simulink model "MSDR_v1.1"  (R2018a)
settings: Solver=ode3  StartTime=0.0  StopTime=21600  FixedStep=0.05
values from neighbouring files (symbols this model uses):
  a_f = -3.22E-5    (= -3.22e-05)    [MSDR_parameters.m]
  a_g = +2.35E-5    (= 2.35e-05)    [MSDR_parameters.m]
  A_s = 1.2245    [MSDR_parameters.m]
  beta = [0.000223, 0.001457, 0.001307, 0.002628, 0.000766, 0.000280]    [MSDR_parameters.m]
  beta_t = sum(beta)    [MSDR_parameters.m]
  ce1 = 1.2471e-07    [MSDR_parameters.m]
  ce2 = 5.3816e-14    [MSDR_parameters.m]
  ce3 = 3.3721e-08    [MSDR_parameters.m]
  Cp_fw = 3200.448e-6    (= 0.003200448)    [MSDR_parameters.m]
  Cp_hr = 0.0021520    (= 0.002152)    [MSDR_parameters.m]
  Cp_p = Cp_s_shx    (= 0.00154912)    [MSDR_parameters.m]
  Cp_s = Cp_s*1e-6    (= 3.588208e-09)    [MSDR_parameters.m]
  Cp_s_shx = 1549.12e-6    (= 0.00154912)    [MSDR_parameters.m]
  Cp_sc = 4761.392e-6    (= 0.004761392)    [MSDR_parameters.m]
  Cp_w = 456.056e-6    (= 0.000456056)    [MSDR_parameters.m]
  D_it = 0.0141478    [MSDR_parameters.m]
  D_ot = 0.015875    [MSDR_parameters.m]
  dHs_dPs = -0.042433622114357    (= -0.0424336221144)    [MSDR_parameters.m]
  eta_hp_isen = 0.861    [MSDR_parameters.m]
  eta_lp_isen = 0.861    [MSDR_parameters.m]
  gamma_I = 5.1135e-2    (= 0.051135)    [MSDR_parameters.m]
  gamma_Xe = 1.1628e-2    (= 0.011628)    [MSDR_parameters.m]
  H_fwh1 = 0.46009    [MSDR_parameters.m]
  h_fwh1 = 0.5927    [MSDR_parameters.m]
  H_fwh2 = 0.6784    [MSDR_parameters.m]
  h_fwh2 = 0.5927    [MSDR_parameters.m]
  H_lp_isen = 958.4*1054.35e-6/0.45359237    (= 2.22774699671)    [MSDR_parameters.m]
  H_nc = 3.2952    [MSDR_parameters.m]
  h_pw = h_s_shx    (= 0.00567446)    [MSDR_parameters.m]
  H_rh = 2.8115    [MSDR_parameters.m]
  h_wb = 13349.334646671E-6    (= 0.0133493346467)    [MSDR_parameters.m]
  h_ws = 5732.378387768E-6    (= 0.00573237838777)    [MSDR_parameters.m]
  h_wsc = 8385.005556375E-6    (= 0.00838500555638)    [MSDR_parameters.m]
  hA_fg = [h_fg*A_fg/2, h_fg*A_fg/2]    [MSDR_parameters.m]
  hA_p_phx1 = h_p_phx*A_p_phx    [MSDR_parameters.m]
  hA_p_phx2 = h_p_phx*A_p_phx    [MSDR_parameters.m]
  hA_p_phx3 = h_p_phx*A_p_phx    [MSDR_parameters.m]
  hA_p_phx4 = h_p_phx*A_p_phx    [MSDR_parameters.m]
  hA_p_phx5 = h_p_phx*A_p_phx    [MSDR_parameters.m]
  hA_p_phx6 = h_p_phx*A_p_phx    [MSDR_parameters.m]
  hA_p_shx1 = h_p_shx*A_p_shx    [MSDR_parameters.m]
  hA_p_shx2 = h_p_shx*A_p_shx    [MSDR_parameters.m]
  hA_p_shx3 = h_p_shx*A_p_shx    [MSDR_parameters.m]
  hA_p_shx4 = h_p_shx*A_p_shx    [MSDR_parameters.m]
  hA_p_shx5 = h_p_shx*A_p_shx    [MSDR_parameters.m]
  hA_p_shx6 = h_p_shx*A_p_shx    [MSDR_parameters.m]
  hA_s_phx1 = h_s_phx*A_s_phx    [MSDR_parameters.m]
  hA_s_phx2 = h_s_phx*A_s_phx    [MSDR_parameters.m]
  hA_s_phx3 = h_s_phx*A_s_phx    [MSDR_parameters.m]
  hA_s_phx4 = h_s_phx*A_s_phx    [MSDR_parameters.m]
  hA_s_phx5 = h_s_phx*A_s_phx    [MSDR_parameters.m]
  hA_s_phx6 = h_s_phx*A_s_phx    [MSDR_parameters.m]
  hA_s_shx1 = h_s_shx*A_s_shx    [MSDR_parameters.m]
  hA_s_shx2 = h_s_shx*A_s_shx    [MSDR_parameters.m]
  hA_s_shx3 = h_s_shx*A_s_shx    [MSDR_parameters.m]
  hA_s_shx4 = h_s_shx*A_s_shx    [MSDR_parameters.m]
  hA_s_shx5 = h_s_shx*A_s_shx    [MSDR_parameters.m]
  hA_s_shx6 = h_s_shx*A_s_shx    [MSDR_parameters.m]
  I_0 = gamma_I*Sig_f_msdr*phi_0/lam_I    (= 4.38204721773e+16)    [MSDR_parameters.m]
  Ifa = [0.25, 0.25]    [MSDR_parameters.m]
  Ifb = [0.25, 0.25]    [MSDR_parameters.m]
  Ig = [0.5, 0.5]    [MSDR_parameters.m]
  K_1 = 11.632248097704855    (= 11.6322480977)    [MSDR_parameters.m]
  K_4 = b(1)    [MSDR_parameters.m]
  K_5 = a(1)    [MSDR_parameters.m]
  K_b = 12.834854076292217    (= 12.8348540763)    [MSDR_parameters.m]
  K_b_hp = 0.1634    [MSDR_parameters.m]
  K_b_lp = 0.2174    [MSDR_parameters.m]
  K_sc = -17.615718797133468    (= -17.6157187971)    [MSDR_parameters.m]
  ka = [0.235, 0.235]    [MSDR_parameters.m]
  kb = [0.235, 0.235]    [MSDR_parameters.m]
  kga = [0.015, 0.015]    [MSDR_parameters.m]
  kgb = [0.015, 0.015]    [MSDR_parameters.m]
  L = 8.5344    [MSDR_parameters.m]
  L_b = 2.3645    [MSDR_parameters.m]
  L_s = 4.723    [MSDR_parameters.m]
  Lam = 2.400E-04    (= 0.00024)    [MSDR_parameters.m]
  lam = [0.0124, 0.0305, 0.111, 0.301, 1.14, 3.01]    [MSDR_parameters.m]
  lam_bubl = 2.0e-2    (= 0.02)    [MSDR_parameters.m]
  lam_I = 2.875e-5    (= 2.875e-05)    [MSDR_parameters.m]
  lam_Xe = 2.0916e-5    (= 2.0916e-05)    [MSDR_parameters.m]
  m_3m = W_3*2    (= 8618.207327)    [MSDR_parameters.m]
  m_fm = W_f*2    (= 9978.96)    [MSDR_parameters.m]
  m_sb = 1717    [MSDR_parameters.m]
  M_stm = 0.018    [MSDR_parameters.m]
  mb_cpb = 2.689619410657651e+00    (= 2.68961941066)    [MSDR_parameters.m]
  mcp_fa = mfa*Cp_f    [MSDR_parameters.m]
  mcp_fb = mfb*Cp_f    [MSDR_parameters.m]
  mcp_g = mg*Cp_g    [MSDR_parameters.m]
  mcp_p_phx1 = Cp_p_phx*mp_phx1    [MSDR_parameters.m]
  mcp_p_phx2 = Cp_p_phx*mp_phx2    [MSDR_parameters.m]
  mcp_p_phx3 = Cp_p_phx*mp_phx3    [MSDR_parameters.m]
  mcp_p_phx4 = Cp_p_phx*mp_phx4    [MSDR_parameters.m]
  mcp_p_phx5 = Cp_p_phx*mp_phx5    [MSDR_parameters.m]
  mcp_p_phx6 = Cp_p_phx*mp_phx6    [MSDR_parameters.m]
  mcp_p_shx1 = Cp_p_shx*mp_shx1    [MSDR_parameters.m]
  mcp_p_shx2 = Cp_p_shx*mp_shx2    [MSDR_parameters.m]
  mcp_p_shx3 = Cp_p_shx*mp_shx3    [MSDR_parameters.m]
  mcp_p_shx4 = Cp_p_shx*mp_shx4    [MSDR_parameters.m]
  mcp_p_shx5 = Cp_p_shx*mp_shx5    [MSDR_parameters.m]
  mcp_p_shx6 = Cp_p_shx*mp_shx6    [MSDR_parameters.m]
  mcp_s_phx1 = Cp_s_phx*ms_phx1    [MSDR_parameters.m]
  mcp_s_phx2 = Cp_s_phx*ms_phx2    [MSDR_parameters.m]
  mcp_s_phx3 = Cp_s_phx*ms_phx3    [MSDR_parameters.m]
  mcp_s_phx4 = Cp_s_phx*ms_phx4    [MSDR_parameters.m]
  mcp_s_phx5 = Cp_s_phx*ms_phx5    [MSDR_parameters.m]
  mcp_s_phx6 = Cp_s_phx*ms_phx6    [MSDR_parameters.m]
  mcp_s_shx1 = Cp_s_shx*ms_shx1    [MSDR_parameters.m]
  mcp_s_shx2 = Cp_s_shx*ms_shx1    [MSDR_parameters.m]
  mcp_s_shx3 = Cp_s_shx*ms_shx1    [MSDR_parameters.m]
  mcp_s_shx4 = Cp_s_shx*ms_shx1    [MSDR_parameters.m]
  mcp_s_shx5 = Cp_s_shx*ms_shx1    [MSDR_parameters.m]
  mcp_s_shx6 = Cp_s_shx*ms_shx1    [MSDR_parameters.m]
  mcp_t_phx1 = Cp_t_phx*mt_phx1    [MSDR_parameters.m]
  mcp_t_phx2 = Cp_t_phx*mt_phx2    [MSDR_parameters.m]
  mcp_t_phx3 = Cp_t_phx*mt_phx3    [MSDR_parameters.m]
  mcp_t_phx4 = Cp_t_phx*mt_phx4    [MSDR_parameters.m]
  mcp_t_phx5 = Cp_t_phx*mt_phx5    [MSDR_parameters.m]
  mcp_t_phx6 = Cp_t_phx*mt_phx6    [MSDR_parameters.m]
  mcp_t_shx1 = Cp_t_phx*mt_shx1    [MSDR_parameters.m]
  ... (+177 more)
undefined symbols (not defined in the file or in its folder): C0, H_rh_table, H_rh_table1, H_rh_table2, H_rhvap_table, H_s_table, H_table, hA_p_thx1, hA_p_thx2, hA_p_thx3, hA_s_thx1, hA_s_thx2, hA_s_thx3, mcp_p_thx1, mcp_p_thx2, mcp_p_thx3, mcp_s_thx1, mcp_s_thx2, mcp_s_thx3, mcp_t_thx1, mcp_t_thx2, mcp_t_thx3, mp_thx1, mp_thx2, mp_thx3, ms_thx1, ms_thx2, ms_thx3, P_nc_table, P_rh_table, P_rh_table1, pres_table, rho_rh_table, rho_table, SV_nc_table, T0_p_thx1, T0_p_thx2, T0_p_thx3, T0_s_thx1, T0_s_thx2, T0_s_thx3, T0_t_thx1, T0_t_thx2, T0_t_thx3, temp_table, u14, Wp_thx1, Wp_thx2
libraries: simulink x13
(part 2 of 6)

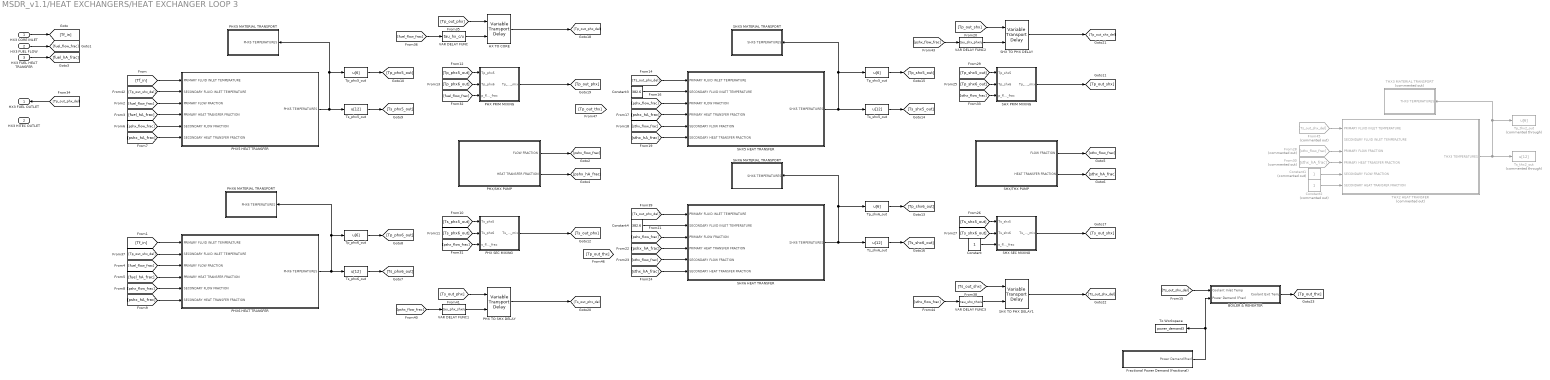
== system MSDR_v1.1/HEAT EXCHANGERS/HEAT EXCHANGER LOOP 3 ==
  HX3 CORE INLET : Inport
  HX3 FUEL FLOW : Inport  Port=2
  HX3 FUEL HEAT TRANSFER : Inport  Port=3
  BOILER & REHEATER : Subsystem
  Constant : Constant
  Constant1 : Constant  Commented=on
  Constant2 : Constant  Commented=on
  Constant3 : Constant  Value=382.6
  Constant4 : Constant  Value=382.6
  Fractional Power Demand (fractional) : Subsystem
  From28 : From  Commented=on  GotoTag=sthx_flow_frac
  From30 : From  Commented=on  GotoTag=sthx_hA_frac
  From45 : From  Commented=on  GotoTag=Ts_out_shx_del
  HX TO CORE : VariableTransportDelay  MaximumDelay=1000000000000  InitialOutput=T0_p_phx5(4)
  PHX PRIM MIXING : Subsystem
  PHX SEC MIXING : Subsystem
  PHX TO SHX DELAY : VariableTransportDelay  MaximumDelay=100000000000  InitialOutput=T0_s_phx5(4)
  PHX/SHX PUMP : Subsystem
  PHX5 HEAT TRANSFER : Subsystem
  PHX5 MATERIAL TRANSPORT : Subsystem
  PHX6 HEAT TRANSFER : Subsystem
  PHX6 MATERIAL TRANSPORT : Subsystem
  SHX PRIM MIXING : Subsystem
  SHX SEC MIXING : Subsystem
  SHX TO PHX DELAY : VariableTransportDelay  MaximumDelay=1000000000000  InitialOutput=T0_p_shx5(4)
  SHX TO PHX DELAY1 : VariableTransportDelay  MaximumDelay=1000000000000  InitialOutput=T0_s_shx5(4)
  SHX/THX PUMP : Subsystem
  SHX5 HEAT TRANSFER : Subsystem
  SHX5 MATERIAL TRANSPORT : Subsystem
  SHX6 HEAT TRANSFER : Subsystem
  SHX6 MATERIAL TRANSPORT : Subsystem
  THX2 HEAT TRANSFER : Subsystem  Commented=on
  THX3 MATERIAL TRANSPORT : Subsystem  Commented=on
  To Workspace : ToWorkspace  VariableName=power_demand3  SampleTime=-1
  Tp_phx5_out : Fcn  Expr=u[6]
  Tp_phx6_out : Fcn  Expr=u[6]
  Tp_shx5_out : Fcn  Expr=u[6]
  Tp_shx6_out : Fcn  Expr=u[6]
  Tp_thx2_out : Fcn  Commented=through  Expr=u[6]
  Ts_phx5_out : Fcn  Expr=u[12]
  Ts_phx6_out : Fcn  Expr=u[12]
  Ts_shx5_out : Fcn  Expr=u[12]
  Ts_shx6_out : Fcn  Expr=u[12]
  Ts_thx2_out : Fcn  Commented=through  Expr=u[12]
  VAR DELAY FUNC : Fcn  Expr=tau_hx_c/u
  VAR DELAY FUNC1 : Fcn  Expr=tau_phx_shx/u
  VAR DELAY FUNC2 : Fcn  Expr=tau_shx_phx/u
  VAR DELAY FUNC3 : Fcn  Expr=tau_shx_thx/u
  HX3 FUEL OUTLET : Outport
  HX3 HITEC OUTLET : Outport  Port=2
  wires:
  HX3 FUEL FLOW/1 -> [fuel_flow_frac]
  HX3 FUEL HEAT TRANSFER/1 -> [fuel_hA_frac]
  HX3 CORE INLET/1 -> [Tf_in]
  [Tp_out_phx_del] -> HX3 FUEL OUTLET/1
  PHX5 HEAT TRANSFER/1(PHX5 TEMPERATURES) -> PHX5 MATERIAL TRANSPORT/1(PHX5 TEMPERATURES), Tp_phx5_out/1, Ts_phx5_out/1
  Tp_phx5_out/1 -> [Tp_phx5_out]
  Ts_phx5_out/1 -> [Ts_phx5_out]
  PHX6 HEAT TRANSFER/1(PHX6 TEMPERATURES) -> PHX6 MATERIAL TRANSPORT/1(PHX6 TEMPERATURES), Tp_phx6_out/1, Ts_phx6_out/1
  Tp_phx6_out/1 -> [Tp_phx6_out]
  Ts_phx6_out/1 -> [Ts_phx6_out]
  PHX/SHX PUMP/2(HEAT TRANSFER FRACTION) -> [pshx_hA_frac]
  [pshx_flow_frac] -> PHX SEC MIXING/3(s_flow_frac)
  [Ts_phx5_out] -> PHX SEC MIXING/1(Ts_phx5)
  PHX/SHX PUMP/1(FLOW FRACTION) -> [pshx_flow_frac]
  [Ts_phx6_out] -> PHX SEC MIXING/2(Ts_phx6)
  PHX SEC MIXING/1(Ts_phx_mix) -> [Ts_out_phx]
  [Tp_phx6_out] -> PHX PRIM MIXING/2(Tp_phx6)
  PHX PRIM MIXING/1(Tp_phx_mix) -> [Tp_out_phx]
  [Tp_phx5_out] -> PHX PRIM MIXING/1(Tp_phx5)
  [fuel_flow_frac] -> PHX PRIM MIXING/3(p_flow_frac)
  Ts_shx5_out/1 -> [Ts_shx5_out]
  Tp_shx5_out/1 -> [Tp_shx5_out]
  SHX5 HEAT TRANSFER/1(SHX5 TEMPERATURES) -> Ts_shx5_out/1, SHX5 MATERIAL TRANSPORT/1(SHX5 TEMPERATURES), Tp_shx5_out/1
  SHX6 HEAT TRANSFER/1(SHX6 TEMPERATURES) -> Ts_shx6_out/1, SHX6 MATERIAL TRANSPORT/1(SHX6 TEMPERATURES), Tp_shx6_out/1
  Ts_shx6_out/1 -> [Ts_shx6_out]
  Tp_shx6_out/1 -> [Tp_shx6_out]
  SHX/THX PUMP/1(FLOW FRACTION) -> [sthx_flow_frac]
  [sthx_flow_frac] -> SHX PRIM MIXING/3(p_flow_frac)
  SHX SEC MIXING/1(Ts_shx_mix) -> [Ts_out_shx]
  SHX/THX PUMP/2(HEAT TRANSFER FRACTION) -> [sthx_hA_frac]
  SHX PRIM MIXING/1(Tp_shx_mix) -> [Tp_out_shx]
  [Ts_shx5_out] -> SHX SEC MIXING/1(Ts_shx5)
  [Tp_shx5_out] -> SHX PRIM MIXING/1(Tp_shx5)
  Constant/1 -> SHX SEC MIXING/3(s_flow_frac)
  [Ts_shx6_out] -> SHX SEC MIXING/2(Ts_shx6)
  [Tp_shx6_out] -> SHX PRIM MIXING/2(Tp_shx6)
  THX2 HEAT TRANSFER/1(THX3 TEMPERATURES) -> THX3 MATERIAL TRANSPORT/1(THX3 TEMPERATURES), Tp_thx2_out/1, Ts_thx2_out/1
  [pshx_hA_frac] -> PHX5 HEAT TRANSFER/6(SECONDARY HEAT TRANSFER FRACTION)
  [Tp_out_shx_del] -> PHX5 HEAT TRANSFER/2(SECONDARY FLUID INLET TEMPERATURE)
  [pshx_flow_frac] -> PHX5 HEAT TRANSFER/5(SECONDARY FLOW FRACTION)
  [fuel_hA_frac] -> PHX5 HEAT TRANSFER/4(PRIMARY HEAT TRANSFER FRACTION)
  [Tf_in] -> PHX5 HEAT TRANSFER/1(PRIMARY FLUID INLET TEMPERATURE)
  [fuel_flow_frac] -> PHX5 HEAT TRANSFER/3(PRIMARY FLOW FRACTION)
  [pshx_flow_frac] -> PHX6 HEAT TRANSFER/5(SECONDARY FLOW FRACTION)
  [fuel_hA_frac] -> PHX6 HEAT TRANSFER/4(PRIMARY HEAT TRANSFER FRACTION)
  [pshx_hA_frac] -> PHX6 HEAT TRANSFER/6(SECONDARY HEAT TRANSFER FRACTION)
  [Tf_in] -> PHX6 HEAT TRANSFER/1(PRIMARY FLUID INLET TEMPERATURE)
  [fuel_flow_frac] -> PHX6 HEAT TRANSFER/3(PRIMARY FLOW FRACTION)
  [Tp_out_shx_del] -> PHX6 HEAT TRANSFER/2(SECONDARY FLUID INLET TEMPERATURE)
  [fuel_flow_frac] -> VAR DELAY FUNC/1
  [Tp_out_phx] -> HX TO CORE/1
  HX TO CORE/1 -> [Tp_out_phx_del]
  VAR DELAY FUNC/1 -> HX TO CORE/2
  PHX TO SHX DELAY/1 -> [Ts_out_phx_del]
  [pshx_flow_frac] -> VAR DELAY FUNC1/1
  VAR DELAY FUNC1/1 -> PHX TO SHX DELAY/2
  [Ts_out_phx] -> PHX TO SHX DELAY/1
  [pshx_flow_frac] -> SHX5 HEAT TRANSFER/3(PRIMARY FLOW FRACTION)
  [pshx_hA_frac] -> SHX5 HEAT TRANSFER/4(PRIMARY HEAT TRANSFER FRACTION)
  [sthx_hA_frac] -> SHX5 HEAT TRANSFER/6(SECONDARY HEAT TRANSFER FRACTION)
  [Ts_out_phx_del] -> SHX5 HEAT TRANSFER/1(PRIMARY FLUID INLET TEMPERATURE)
  [sthx_flow_frac] -> SHX5 HEAT TRANSFER/5(SECONDARY FLOW FRACTION)
  [sthx_hA_frac] -> SHX6 HEAT TRANSFER/6(SECONDARY HEAT TRANSFER FRACTION)
  [pshx_hA_frac] -> SHX6 HEAT TRANSFER/4(PRIMARY HEAT TRANSFER FRACTION)
  [pshx_flow_frac] -> SHX6 HEAT TRANSFER/3(PRIMARY FLOW FRACTION)
  [sthx_flow_frac] -> SHX6 HEAT TRANSFER/5(SECONDARY FLOW FRACTION)
  [Ts_out_phx_del] -> SHX6 HEAT TRANSFER/1(PRIMARY FLUID INLET TEMPERATURE)
  VAR DELAY FUNC2/1 -> SHX TO PHX DELAY/2
  [Tp_out_shx] -> SHX TO PHX DELAY/1
  [pshx_flow_frac] -> VAR DELAY FUNC2/1
  SHX TO PHX DELAY/1 -> [Tp_out_shx_del]
  [Ts_out_shx] -> SHX TO PHX DELAY1/1
  SHX TO PHX DELAY1/1 -> [Ts_out_shx_del]
  [sthx_flow_frac] -> VAR DELAY FUNC3/1
  VAR DELAY FUNC3/1 -> SHX TO PHX DELAY1/2
  Constant1/1 -> THX2 HEAT TRANSFER/5(SECONDARY FLOW FRACTION)
  Constant2/1 -> THX2 HEAT TRANSFER/6(SECONDARY HEAT TRANSFER FRACTION)
  From45/1 -> THX2 HEAT TRANSFER/1(PRIMARY FLUID INLET TEMPERATURE)
  From28/1 -> THX2 HEAT TRANSFER/3(PRIMARY FLOW FRACTION)
  From30/1 -> THX2 HEAT TRANSFER/4(PRIMARY HEAT TRANSFER FRACTION)
  BOILER & REHEATER/1(Coolant Exit Temp) -> [Tp_out_thx]
  [Ts_out_shx_del] -> BOILER & REHEATER/1(Coolant Inlet Temp)
  Fractional Power Demand (fractional)/1(Power Demand(frac)) -> To Workspace/1, BOILER & REHEATER/2(Power Demand (Frac))
  Constant3/1 -> SHX5 HEAT TRANSFER/2(SECONDARY FLUID INLET TEMPERATURE)
  Constant4/1 -> SHX6 HEAT TRANSFER/2(SECONDARY FLUID INLET TEMPERATURE)

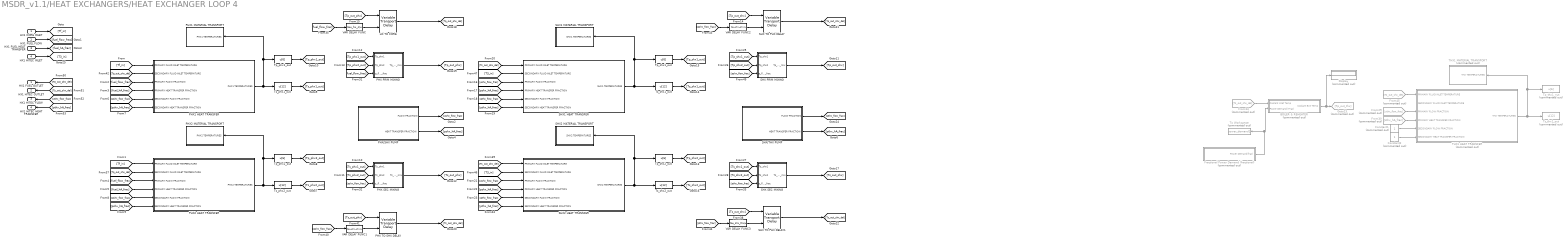
== system MSDR_v1.1/HEAT EXCHANGERS/HEAT EXCHANGER LOOP 4 ==
  HX1 CORE INLET : Inport
  HX1 FUEL FLOW : Inport  Port=2
  HX1 FUEL HEAT TRANSFER : Inport  Port=3
  HX1 HITEC INLET : Inport  Port=4
  BOILER & REHEATER : Subsystem  Commented=on
  Constant1 : Constant  Commented=on
  Constant2 : Constant  Commented=on
  Display : Display  Commented=on
  Fractional Power Demand (fractional) : Subsystem  Commented=on
  From29 : From  Commented=on  GotoTag=sthx_flow_frac
  From30 : From  Commented=on  GotoTag=sthx_hA_frac
  From34 : From  Commented=on  GotoTag=Ts_out_shx_del
  From45 : From  Commented=on  GotoTag=Ts_out_shx_del
  Goto23 : Goto  Commented=on  GotoTag=Tp_out_thx
  HX TO CORE : VariableTransportDelay  MaximumDelay=1000000000000  InitialOutput=T0_p_phx1(4)
  PHX PRIM MIXING : Subsystem
  PHX SEC MIXING : Subsystem
  PHX TO SHX DELAY : VariableTransportDelay  MaximumDelay=100000000000  InitialOutput=T0_s_phx1(4)
  PHX/SHX PUMP : Subsystem
  PHX1 HEAT TRANSFER : Subsystem
  PHX1 MATERIAL TRANSPORT : Subsystem
  PHX2 HEAT TRANSFER : Subsystem
  PHX2 MATERIAL TRANSPORT : Subsystem
  SHX PRIM MIXING : Subsystem
  SHX SEC MIXING : Subsystem
  SHX TO PHX DELAY : VariableTransportDelay  MaximumDelay=1000000000000  InitialOutput=T0_p_shx1(4)
  SHX TO PHX DELAY1 : VariableTransportDelay  MaximumDelay=1000000000000  InitialOutput=T0_s_shx1(4)
  SHX/THX PUMP : Subsystem
  SHX1 HEAT TRANSFER : Subsystem
  SHX1 MATERIAL TRANSPORT : Subsystem
  SHX2 HEAT TRANSFER : Subsystem
  SHX2 MATERIAL TRANSPORT : Subsystem
  THX1 HEAT TRANSFER : Subsystem  Commented=on
  THX1 MATERIAL TRANSPORT : Subsystem  Commented=on
  To Workspace : ToWorkspace  Commented=on  VariableName=power_demand1  SampleTime=-1
  Tp_phx1_out : Fcn  Expr=u[6]
  Tp_phx2_out : Fcn  Expr=u[6]
  Tp_shx1_out : Fcn  Expr=u[6]
  Tp_shx2_out : Fcn  Expr=u[6]
  Tp_thx1_out : Fcn  Commented=on  Expr=u[6]
  Ts_phx1_out : Fcn  Expr=u[12]
  Ts_phx2_out : Fcn  Expr=u[12]
  Ts_shx1_out : Fcn  Expr=u[12]
  Ts_shx2_out : Fcn  Expr=u[12]
  Ts_thx1_out : Fcn  Commented=on  Expr=u[12]
  VAR DELAY FUNC : Fcn  Expr=tau_hx_c/u
  VAR DELAY FUNC1 : Fcn  Expr=tau_phx_shx/u
  VAR DELAY FUNC2 : Fcn  Expr=tau_shx_phx/u
  VAR DELAY FUNC3 : Fcn  Expr=tau_shx_thx/u
  HX1 FUEL OUTLET : Outport
  HX1 HITEC OUTLET : Outport  Port=2
  HX1 HITEC FLOW : Outport  Port=3
  HX1 HITEC HEAT TRANSFER : Outport  Port=4
  wires:
  PHX1 HEAT TRANSFER/1(PHX1 TEMPERATURES) -> PHX1 MATERIAL TRANSPORT/1(PHX1 TEMPERATURES), Tp_phx1_out/1, Ts_phx1_out/1
  THX1 HEAT TRANSFER/1(THX TEMPERATURES) -> THX1 MATERIAL TRANSPORT/1(THX TEMPERATURES), Tp_thx1_out/1, Ts_thx1_out/1
  SHX1 HEAT TRANSFER/1(SHX1 TEMPERATURES) -> Ts_shx1_out/1, Tp_shx1_out/1, SHX1 MATERIAL TRANSPORT/1(SHX1 TEMPERATURES)
  PHX2 HEAT TRANSFER/1(PHX2 TEMPERATURES) -> PHX2 MATERIAL TRANSPORT/1(PHX2 TEMPERATURES), Tp_phx2_out/1, Ts_phx2_out/1
  SHX2 HEAT TRANSFER/1(SHX2 TEMPERATURES) -> Ts_shx2_out/1, SHX2 MATERIAL TRANSPORT/1(SHX2 TEMPERATURES), Tp_shx2_out/1
  HX1 CORE INLET/1 -> [Tf_in]
  [Tf_in] -> PHX1 HEAT TRANSFER/1(PRIMARY FLUID INLET TEMPERATURE)
  [Tf_in] -> PHX2 HEAT TRANSFER/1(PRIMARY FLUID INLET TEMPERATURE)
  HX1 FUEL FLOW/1 -> [fuel_flow_frac]
  HX1 FUEL HEAT TRANSFER/1 -> [fuel_hA_frac]
  [fuel_flow_frac] -> PHX1 HEAT TRANSFER/3(PRIMARY FLOW FRACTION)
  [fuel_hA_frac] -> PHX1 HEAT TRANSFER/4(PRIMARY HEAT TRANSFER FRACTION)
  [fuel_flow_frac] -> PHX2 HEAT TRANSFER/3(PRIMARY FLOW FRACTION)
  [fuel_hA_frac] -> PHX2 HEAT TRANSFER/4(PRIMARY HEAT TRANSFER FRACTION)
  PHX/SHX PUMP/2(HEAT TRANSFER FRACTION) -> [pshx_hA_frac]
  PHX/SHX PUMP/1(FLOW FRACTION) -> [pshx_flow_frac]
  SHX/THX PUMP/1(FLOW FRACTION) -> [pthx_flow_frac]
  SHX/THX PUMP/2(HEAT TRANSFER FRACTION) -> [pthx_hA_frac]
  Ts_phx2_out/1 -> [Ts_phx2_out]
  Tp_phx2_out/1 -> [Tp_phx2_out]
  Tp_phx1_out/1 -> [Tp_phx1_out]
  Ts_phx1_out/1 -> [Ts_phx1_out]
  [pshx_flow_frac] -> PHX1 HEAT TRANSFER/5(SECONDARY FLOW FRACTION)
  [pshx_hA_frac] -> PHX1 HEAT TRANSFER/6(SECONDARY HEAT TRANSFER FRACTION)
  [pshx_flow_frac] -> PHX2 HEAT TRANSFER/5(SECONDARY FLOW FRACTION)
  [pshx_hA_frac] -> PHX2 HEAT TRANSFER/6(SECONDARY HEAT TRANSFER FRACTION)
  [Tp_phx1_out] -> PHX PRIM MIXING/1(Tp_phx1)
  [Tp_phx2_out] -> PHX PRIM MIXING/2(Tp_phx2)
  PHX PRIM MIXING/1(Tp_phx_mix) -> [Tp_out_phx]
  [Ts_out_phx_del] -> SHX1 HEAT TRANSFER/1(PRIMARY FLUID INLET TEMPERATURE)
  [pshx_flow_frac] -> SHX1 HEAT TRANSFER/3(PRIMARY FLOW FRACTION)
  [pshx_hA_frac] -> SHX1 HEAT TRANSFER/4(PRIMARY HEAT TRANSFER FRACTION)
  [pthx_flow_frac] -> SHX1 HEAT TRANSFER/5(SECONDARY FLOW FRACTION)
  [pthx_hA_frac] -> SHX1 HEAT TRANSFER/6(SECONDARY HEAT TRANSFER FRACTION)
  [Ts_out_phx_del] -> SHX2 HEAT TRANSFER/1(PRIMARY FLUID INLET TEMPERATURE)
  [pshx_flow_frac] -> SHX2 HEAT TRANSFER/3(PRIMARY FLOW FRACTION)
  [pshx_hA_frac] -> SHX2 HEAT TRANSFER/4(PRIMARY HEAT TRANSFER FRACTION)
  [pthx_flow_frac] -> SHX2 HEAT TRANSFER/5(SECONDARY FLOW FRACTION)
  [pthx_hA_frac] -> SHX2 HEAT TRANSFER/6(SECONDARY HEAT TRANSFER FRACTION)
  Tp_shx1_out/1 -> [Tp_shx1_out]
  Tp_shx2_out/1 -> [Tp_shx2_out]
  Ts_shx1_out/1 -> [Ts_shx1_out]
  Ts_shx2_out/1 -> [Ts_shx2_out]
  From29/1 -> THX1 HEAT TRANSFER/3(PRIMARY FLOW FRACTION)
  From30/1 -> THX1 HEAT TRANSFER/4(PRIMARY HEAT TRANSFER FRACTION)
  [fuel_flow_frac] -> PHX PRIM MIXING/3(p_flow_frac)
  [pshx_flow_frac] -> PHX SEC MIXING/3(s_flow_frac)
  [Ts_phx2_out] -> PHX SEC MIXING/2(Ts_phx2)
  [Ts_phx1_out] -> PHX SEC MIXING/1(Ts_phx1)
  PHX SEC MIXING/1(Ts_phx_mix) -> [Ts_out_phx]
  [Tp_shx2_out] -> SHX PRIM MIXING/2(Tp_shx2)
  [Tp_shx1_out] -> SHX PRIM MIXING/1(Tp_shx1)
  SHX PRIM MIXING/1(Tp_shx_mix) -> [Tp_out_shx]
  From45/1 -> THX1 HEAT TRANSFER/1(PRIMARY FLUID INLET TEMPERATURE)
  [Ts_shx1_out] -> SHX SEC MIXING/1(Ts_shx1)
  SHX SEC MIXING/1(Ts_shx_mix) -> [Ts_out_shx]
  [Ts_shx2_out] -> SHX SEC MIXING/2(Ts_shx2)
  [pthx_flow_frac] -> SHX SEC MIXING/3(s_flow_frac)
  Constant1/1 -> THX1 HEAT TRANSFER/5(SECONDARY FLOW FRACTION)
  Constant2/1 -> THX1 HEAT TRANSFER/6(SECONDARY HEAT TRANSFER FRACTION)
  [Tp_out_shx_del] -> PHX1 HEAT TRANSFER/2(SECONDARY FLUID INLET TEMPERATURE)
  [Tp_out_shx_del] -> PHX2 HEAT TRANSFER/2(SECONDARY FLUID INLET TEMPERATURE)
  VAR DELAY FUNC/1 -> HX TO CORE/2
  [Tp_out_phx] -> HX TO CORE/1
  [fuel_flow_frac] -> VAR DELAY FUNC/1
  HX TO CORE/1 -> [Tp_out_phx_del]
  VAR DELAY FUNC1/1 -> PHX TO SHX DELAY/2
  PHX TO SHX DELAY/1 -> [Ts_out_phx_del]
  [Ts_out_phx] -> PHX TO SHX DELAY/1
  [pshx_flow_frac] -> VAR DELAY FUNC1/1
  VAR DELAY FUNC2/1 -> SHX TO PHX DELAY/2
  SHX TO PHX DELAY/1 -> [Tp_out_shx_del]
  [pshx_flow_frac] -> VAR DELAY FUNC2/1
  [Tp_out_shx] -> SHX TO PHX DELAY/1
  [Ts_out_shx] -> SHX TO PHX DELAY1/1
  [pthx_flow_frac] -> VAR DELAY FUNC3/1
  SHX TO PHX DELAY1/1 -> [Ts_out_shx_del]
  VAR DELAY FUNC3/1 -> SHX TO PHX DELAY1/2
  Fractional Power Demand (fractional)/1(Power Demand(frac)) -> BOILER & REHEATER/2(Power Demand (Frac)), To Workspace/1
  From34/1 -> BOILER & REHEATER/1(Coolant Inlet Temp)
  BOILER & REHEATER/1(Coolant Exit Temp) -> Display/1, Goto23/1
  [T3_in] -> SHX1 HEAT TRANSFER/2(SECONDARY FLUID INLET TEMPERATURE)
  [T3_in] -> SHX2 HEAT TRANSFER/2(SECONDARY FLUID INLET TEMPERATURE)
  HX1 HITEC INLET/1 -> [T3_in]
  [pshx_flow_frac] -> SHX PRIM MIXING/3(p_flow_frac)
  [pthx_hA_frac] -> HX1 HITEC HEAT TRANSFER/1
  [pthx_flow_frac] -> HX1 HITEC FLOW/1
  [Ts_out_shx_del] -> HX1 HITEC OUTLET/1
  [Tp_out_phx_del] -> HX1 FUEL OUTLET/1

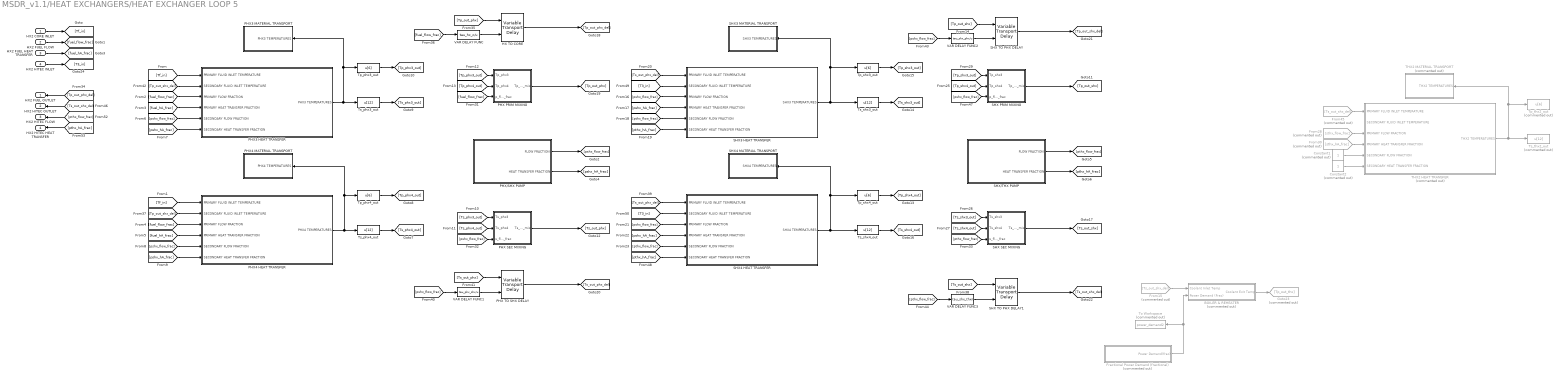
== system MSDR_v1.1/HEAT EXCHANGERS/HEAT EXCHANGER LOOP 5 ==
  HX2 CORE INLET : Inport
  HX2 FUEL FLOW : Inport  Port=2
  HX2 FUEL HEAT TRANSFER : Inport  Port=3
  HX2 HITEC INLET : Inport  Port=4
  BOILER & REHEATER : Subsystem  Commented=on
  Constant1 : Constant  Commented=on
  Constant2 : Constant  Commented=on
  Fractional Power Demand (fractional) : Subsystem  Commented=on
  From15 : From  Commented=on  GotoTag=Ts_out_shx_del
  From28 : From  Commented=on  GotoTag=sthx_flow_frac
  From30 : From  Commented=on  GotoTag=sthx_hA_frac
  From45 : From  Commented=on  GotoTag=Ts_out_shx_del
  Goto23 : Goto  Commented=on  GotoTag=Tp_out_thx
  HX TO CORE : VariableTransportDelay  MaximumDelay=1000000000000  InitialOutput=T0_p_phx3(4)
  PHX PRIM MIXING : Subsystem
  PHX SEC MIXING : Subsystem
  PHX TO SHX DELAY : VariableTransportDelay  MaximumDelay=100000000000  InitialOutput=T0_s_phx3(4)
  PHX/SHX PUMP : Subsystem
  PHX3 HEAT TRANSFER : Subsystem
  PHX3 MATERIAL TRANSPORT : Subsystem
  PHX4 HEAT TRANSFER : Subsystem
  PHX4 MATERIAL TRANSPORT : Subsystem
  SHX PRIM MIXING : Subsystem
  SHX SEC MIXING : Subsystem
  SHX TO PHX DELAY : VariableTransportDelay  MaximumDelay=1000000000000  InitialOutput=T0_p_shx3(4)
  SHX TO PHX DELAY1 : VariableTransportDelay  MaximumDelay=1000000000000  InitialOutput=T0_s_shx3(4)
  SHX/THX PUMP : Subsystem
  SHX3 HEAT TRANSFER : Subsystem
  SHX3 MATERIAL TRANSPORT : Subsystem
  SHX4 HEAT TRANSFER : Subsystem
  SHX4 MATERIAL TRANSPORT : Subsystem
  THX2 HEAT TRANSFER : Subsystem  Commented=on
  THX2 MATERIAL TRANSPORT : Subsystem  Commented=on
  To Workspace : ToWorkspace  Commented=on  VariableName=power_demand2  SampleTime=-1
  Tp_phx3_out : Fcn  Expr=u[6]
  Tp_phx4_out : Fcn  Expr=u[6]
  Tp_shx3_out : Fcn  Expr=u[6]
  Tp_shx4_out : Fcn  Expr=u[6]
  Tp_thx2_out : Fcn  Commented=on  Expr=u[6]
  Ts_phx3_out : Fcn  Expr=u[12]
  Ts_phx4_out : Fcn  Expr=u[12]
  Ts_shx3_out : Fcn  Expr=u[12]
  Ts_shx4_out : Fcn  Expr=u[12]
  Ts_thx2_out : Fcn  Commented=on  Expr=u[12]
  VAR DELAY FUNC : Fcn  Expr=tau_hx_c/u
  VAR DELAY FUNC1 : Fcn  Expr=tau_phx_shx/u
  VAR DELAY FUNC2 : Fcn  Expr=tau_shx_phx/u
  VAR DELAY FUNC3 : Fcn  Expr=tau_shx_thx/u
  HX2 FUEL OUTLET : Outport
  HX2 HITEC OUTLET : Outport  Port=2
  HX2 HITEC FLOW : Outport  Port=3
  HX2 HITEC HEAT TRANSFER : Outport  Port=4
  wires:
  [Tp_out_phx_del] -> HX2 FUEL OUTLET/1
  HX2 CORE INLET/1 -> [Tf_in]
  HX2 FUEL HEAT TRANSFER/1 -> [fuel_hA_frac]
  HX2 FUEL FLOW/1 -> [fuel_flow_frac]
  Tp_phx3_out/1 -> [Tp_phx3_out]
  PHX3 HEAT TRANSFER/1(PHX3 TEMPERATURES) -> PHX3 MATERIAL TRANSPORT/1(PHX3 TEMPERATURES), Tp_phx3_out/1, Ts_phx3_out/1
  Ts_phx3_out/1 -> [Ts_phx3_out]
  Tp_phx4_out/1 -> [Tp_phx4_out]
  Ts_phx4_out/1 -> [Ts_phx4_out]
  PHX4 HEAT TRANSFER/1(PHX4 TEMPERATURES) -> PHX4 MATERIAL TRANSPORT/1(PHX4 TEMPERATURES), Tp_phx4_out/1, Ts_phx4_out/1
  Tp_shx3_out/1 -> [Tp_shx3_out]
  Ts_shx3_out/1 -> [Ts_shx3_out]
  SHX3 HEAT TRANSFER/1(SHX3 TEMPERATURES) -> Ts_shx3_out/1, SHX3 MATERIAL TRANSPORT/1(SHX3 TEMPERATURES), Tp_shx3_out/1
  [Tp_phx3_out] -> PHX PRIM MIXING/1(Tp_phx3)
  [fuel_flow_frac] -> PHX PRIM MIXING/3(p_flow_frac)
  [Ts_phx3_out] -> PHX SEC MIXING/1(Ts_phx3)
  [Ts_phx4_out] -> PHX SEC MIXING/2(Ts_phx4)
  [Tp_phx4_out] -> PHX PRIM MIXING/2(Tp_phx4)
  PHX SEC MIXING/1(Ts_phx_mix) -> [Ts_out_phx]
  PHX/SHX PUMP/1(FLOW FRACTION) -> [pshx_flow_frac]
  PHX PRIM MIXING/1(Tp_phx_mix) -> [Tp_out_phx]
  [pshx_flow_frac] -> PHX SEC MIXING/3(s_flow_frac)
  PHX/SHX PUMP/2(HEAT TRANSFER FRACTION) -> [pshx_hA_frac]
  Tp_shx4_out/1 -> [Tp_shx4_out]
  SHX4 HEAT TRANSFER/1(SHX4 TEMPERATURES) -> Ts_shx4_out/1, SHX4 MATERIAL TRANSPORT/1(SHX4 TEMPERATURES), Tp_shx4_out/1
  Ts_shx4_out/1 -> [Ts_shx4_out]
  [Tp_shx3_out] -> SHX PRIM MIXING/1(Tp_shx3)
  [Ts_shx4_out] -> SHX SEC MIXING/2(Ts_shx4)
  [Ts_shx3_out] -> SHX SEC MIXING/1(Ts_shx3)
  [Tp_shx4_out] -> SHX PRIM MIXING/2(Tp_shx4)
  SHX/THX PUMP/2(HEAT TRANSFER FRACTION) -> [pthx_hA_frac]
  SHX SEC MIXING/1(Ts_shx_mix) -> [Ts_out_shx]
  SHX PRIM MIXING/1(Tp_shx_mix) -> [Tp_out_shx]
  SHX/THX PUMP/1(FLOW FRACTION) -> [pthx_flow_frac]
  [pthx_flow_frac] -> SHX SEC MIXING/3(s_flow_frac)
  THX2 HEAT TRANSFER/1(THX2 TEMPERATURES) -> THX2 MATERIAL TRANSPORT/1(THX2 TEMPERATURES), Tp_thx2_out/1, Ts_thx2_out/1
  [fuel_hA_frac] -> PHX3 HEAT TRANSFER/4(PRIMARY HEAT TRANSFER FRACTION)
  [Tp_out_shx_del] -> PHX3 HEAT TRANSFER/2(SECONDARY FLUID INLET TEMPERATURE)
  [pshx_hA_frac] -> PHX3 HEAT TRANSFER/6(SECONDARY HEAT TRANSFER FRACTION)
  [Tf_in] -> PHX3 HEAT TRANSFER/1(PRIMARY FLUID INLET TEMPERATURE)
  [pshx_flow_frac] -> PHX3 HEAT TRANSFER/5(SECONDARY FLOW FRACTION)
  [fuel_flow_frac] -> PHX3 HEAT TRANSFER/3(PRIMARY FLOW FRACTION)
  [Tp_out_shx_del] -> PHX4 HEAT TRANSFER/2(SECONDARY FLUID INLET TEMPERATURE)
  [pshx_flow_frac] -> PHX4 HEAT TRANSFER/5(SECONDARY FLOW FRACTION)
  [fuel_flow_frac] -> PHX4 HEAT TRANSFER/3(PRIMARY FLOW FRACTION)
  [Tf_in] -> PHX4 HEAT TRANSFER/1(PRIMARY FLUID INLET TEMPERATURE)
  [pshx_hA_frac] -> PHX4 HEAT TRANSFER/6(SECONDARY HEAT TRANSFER FRACTION)
  [fuel_hA_frac] -> PHX4 HEAT TRANSFER/4(PRIMARY HEAT TRANSFER FRACTION)
  VAR DELAY FUNC/1 -> HX TO CORE/2
  HX TO CORE/1 -> [Tp_out_phx_del]
  [Tp_out_phx] -> HX TO CORE/1
  [fuel_flow_frac] -> VAR DELAY FUNC/1
  [Ts_out_phx] -> PHX TO SHX DELAY/1
  [pshx_flow_frac] -> VAR DELAY FUNC1/1
  VAR DELAY FUNC1/1 -> PHX TO SHX DELAY/2
  PHX TO SHX DELAY/1 -> [Ts_out_phx_del]
  [pthx_flow_frac] -> SHX3 HEAT TRANSFER/5(SECONDARY FLOW FRACTION)
  [pthx_hA_frac] -> SHX3 HEAT TRANSFER/6(SECONDARY HEAT TRANSFER FRACTION)
  [pshx_hA_frac] -> SHX3 HEAT TRANSFER/4(PRIMARY HEAT TRANSFER FRACTION)
  [Ts_out_phx_del] -> SHX3 HEAT TRANSFER/1(PRIMARY FLUID INLET TEMPERATURE)
  [pshx_flow_frac] -> SHX3 HEAT TRANSFER/3(PRIMARY FLOW FRACTION)
  [pthx_hA_frac] -> SHX4 HEAT TRANSFER/6(SECONDARY HEAT TRANSFER FRACTION)
  [pthx_flow_frac] -> SHX4 HEAT TRANSFER/5(SECONDARY FLOW FRACTION)
  [pshx_hA_frac] -> SHX4 HEAT TRANSFER/4(PRIMARY HEAT TRANSFER FRACTION)
  [pshx_flow_frac] -> SHX4 HEAT TRANSFER/3(PRIMARY FLOW FRACTION)
  [Ts_out_phx_del] -> SHX4 HEAT TRANSFER/1(PRIMARY FLUID INLET TEMPERATURE)
  [Tp_out_shx] -> SHX TO PHX DELAY/1
  [pshx_flow_frac] -> VAR DELAY FUNC2/1
  SHX TO PHX DELAY/1 -> [Tp_out_shx_del]
  VAR DELAY FUNC2/1 -> SHX TO PHX DELAY/2
  VAR DELAY FUNC3/1 -> SHX TO PHX DELAY1/2
  SHX TO PHX DELAY1/1 -> [Ts_out_shx_del]
  [Ts_out_shx] -> SHX TO PHX DELAY1/1
  [pthx_flow_frac] -> VAR DELAY FUNC3/1
  From30/1 -> THX2 HEAT TRANSFER/4(PRIMARY HEAT TRANSFER FRACTION)
  From45/1 -> THX2 HEAT TRANSFER/1(PRIMARY FLUID INLET TEMPERATURE)
  Constant1/1 -> THX2 HEAT TRANSFER/5(SECONDARY FLOW FRACTION)
  Constant2/1 -> THX2 HEAT TRANSFER/6(SECONDARY HEAT TRANSFER FRACTION)
  From28/1 -> THX2 HEAT TRANSFER/3(PRIMARY FLOW FRACTION)
  BOILER & REHEATER/1(Coolant Exit Temp) -> Goto23/1
  From15/1 -> BOILER & REHEATER/1(Coolant Inlet Temp)
  Fractional Power Demand (fractional)/1(Power Demand(frac)) -> BOILER & REHEATER/2(Power Demand (Frac)), To Workspace/1
  [T3_in] -> SHX3 HEAT TRANSFER/2(SECONDARY FLUID INLET TEMPERATURE)
  [T3_in] -> SHX4 HEAT TRANSFER/2(SECONDARY FLUID INLET TEMPERATURE)
  HX2 HITEC INLET/1 -> [T3_in]
  [Ts_out_shx_del] -> HX2 HITEC OUTLET/1
  [pshx_flow_frac] -> SHX PRIM MIXING/3(p_flow_frac)
  [pthx_flow_frac] -> HX2 HITEC FLOW/1
  [pthx_hA_frac] -> HX2 HITEC HEAT TRANSFER/1

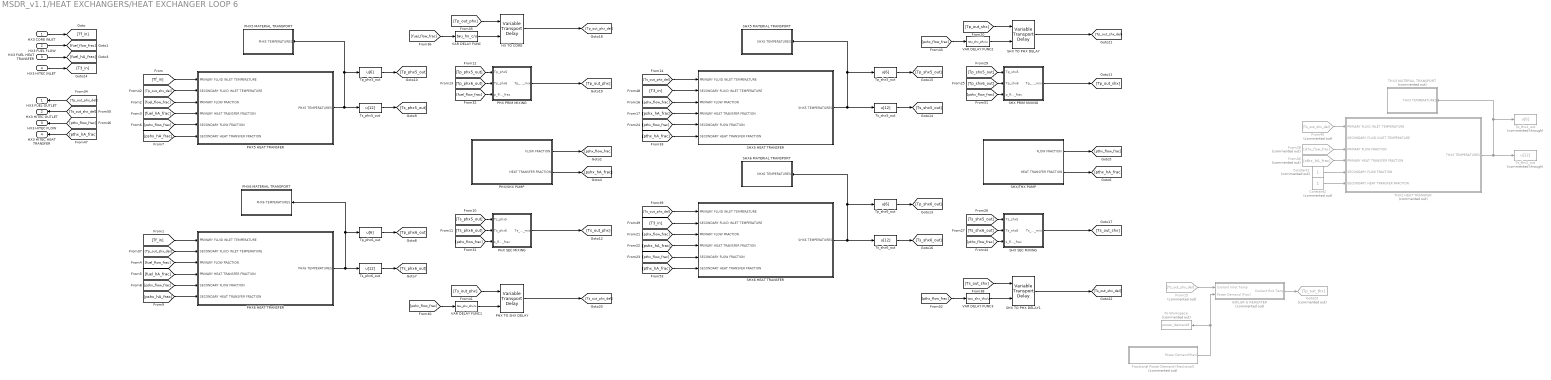
== system MSDR_v1.1/HEAT EXCHANGERS/HEAT EXCHANGER LOOP 6 ==
  HX3 CORE INLET : Inport
  HX3 FUEL FLOW : Inport  Port=2
  HX3 FUEL HEAT TRANSFER : Inport  Port=3
  HX3 HITEC INLET : Inport  Port=4
  BOILER & REHEATER : Subsystem  Commented=on
  Constant1 : Constant  Commented=on
  Constant2 : Constant  Commented=on
  Fractional Power Demand (fractional) : Subsystem  Commented=on
  From15 : From  Commented=on  GotoTag=Ts_out_shx_del
  From28 : From  Commented=on  GotoTag=sthx_flow_frac
  From30 : From  Commented=on  GotoTag=sthx_hA_frac
  From45 : From  Commented=on  GotoTag=Ts_out_shx_del
  Goto23 : Goto  Commented=on  GotoTag=Tp_out_thx
  HX TO CORE : VariableTransportDelay  MaximumDelay=1000000000000  InitialOutput=T0_p_phx5(4)
  PHX PRIM MIXING : Subsystem
  PHX SEC MIXING : Subsystem
  PHX TO SHX DELAY : VariableTransportDelay  MaximumDelay=100000000000  InitialOutput=T0_s_phx5(4)
  PHX/SHX PUMP : Subsystem
  PHX5 HEAT TRANSFER : Subsystem
  PHX5 MATERIAL TRANSPORT : Subsystem
  PHX6 HEAT TRANSFER : Subsystem
  PHX6 MATERIAL TRANSPORT : Subsystem
  SHX PRIM MIXING : Subsystem
  SHX SEC MIXING : Subsystem
  SHX TO PHX DELAY : VariableTransportDelay  MaximumDelay=1000000000000  InitialOutput=T0_p_shx5(4)
  SHX TO PHX DELAY1 : VariableTransportDelay  MaximumDelay=1000000000000  InitialOutput=T0_s_shx5(4)
  SHX/THX PUMP : Subsystem
  SHX5 HEAT TRANSFER : Subsystem
  SHX5 MATERIAL TRANSPORT : Subsystem
  SHX6 HEAT TRANSFER : Subsystem
  SHX6 MATERIAL TRANSPORT : Subsystem
  THX2 HEAT TRANSFER : Subsystem  Commented=on
  THX3 MATERIAL TRANSPORT : Subsystem  Commented=on
  To Workspace : ToWorkspace  Commented=on  VariableName=power_demand3  SampleTime=-1
  Tp_phx5_out : Fcn  Expr=u[6]
  Tp_phx6_out : Fcn  Expr=u[6]
  Tp_shx5_out : Fcn  Expr=u[6]
  Tp_shx6_out : Fcn  Expr=u[6]
  Tp_thx2_out : Fcn  Commented=through  Expr=u[6]
  Ts_phx5_out : Fcn  Expr=u[12]
  Ts_phx6_out : Fcn  Expr=u[12]
  Ts_shx5_out : Fcn  Expr=u[12]
  Ts_shx6_out : Fcn  Expr=u[12]
  Ts_thx2_out : Fcn  Commented=through  Expr=u[12]
  VAR DELAY FUNC : Fcn  Expr=tau_hx_c/u
  VAR DELAY FUNC1 : Fcn  Expr=tau_phx_shx/u
  VAR DELAY FUNC2 : Fcn  Expr=tau_shx_phx/u
  VAR DELAY FUNC3 : Fcn  Expr=tau_shx_thx/u
  HX3 FUEL OUTLET : Outport
  HX3 HITEC OUTLET : Outport  Port=2
  HX3 HITEC FLOW : Outport  Port=3
  HX3 HITEC HEAT TRANSFER : Outport  Port=4
  wires:
  HX3 FUEL FLOW/1 -> [fuel_flow_frac]
  HX3 FUEL HEAT TRANSFER/1 -> [fuel_hA_frac]
  HX3 CORE INLET/1 -> [Tf_in]
  [Tp_out_phx_del] -> HX3 FUEL OUTLET/1
  PHX5 HEAT TRANSFER/1(PHX5 TEMPERATURES) -> PHX5 MATERIAL TRANSPORT/1(PHX5 TEMPERATURES), Tp_phx5_out/1, Ts_phx5_out/1
  Tp_phx5_out/1 -> [Tp_phx5_out]
  Ts_phx5_out/1 -> [Ts_phx5_out]
  PHX6 HEAT TRANSFER/1(PHX6 TEMPERATURES) -> PHX6 MATERIAL TRANSPORT/1(PHX6 TEMPERATURES), Tp_phx6_out/1, Ts_phx6_out/1
  Tp_phx6_out/1 -> [Tp_phx6_out]
  Ts_phx6_out/1 -> [Ts_phx6_out]
  PHX/SHX PUMP/2(HEAT TRANSFER FRACTION) -> [pshx_hA_frac]
  [pshx_flow_frac] -> PHX SEC MIXING/3(s_flow_frac)
  [Ts_phx5_out] -> PHX SEC MIXING/1(Ts_phx5)
  PHX/SHX PUMP/1(FLOW FRACTION) -> [pshx_flow_frac]
  [Ts_phx6_out] -> PHX SEC MIXING/2(Ts_phx6)
  PHX SEC MIXING/1(Ts_phx_mix) -> [Ts_out_phx]
  [Tp_phx6_out] -> PHX PRIM MIXING/2(Tp_phx6)
  PHX PRIM MIXING/1(Tp_phx_mix) -> [Tp_out_phx]
  [Tp_phx5_out] -> PHX PRIM MIXING/1(Tp_phx5)
  [fuel_flow_frac] -> PHX PRIM MIXING/3(p_flow_frac)
  Ts_shx5_out/1 -> [Ts_shx5_out]
  Tp_shx5_out/1 -> [Tp_shx5_out]
  SHX5 HEAT TRANSFER/1(SHX5 TEMPERATURES) -> Ts_shx5_out/1, SHX5 MATERIAL TRANSPORT/1(SHX5 TEMPERATURES), Tp_shx5_out/1
  SHX6 HEAT TRANSFER/1(SHX6 TEMPERATURES) -> Ts_shx6_out/1, SHX6 MATERIAL TRANSPORT/1(SHX6 TEMPERATURES), Tp_shx6_out/1
  Ts_shx6_out/1 -> [Ts_shx6_out]
  Tp_shx6_out/1 -> [Tp_shx6_out]
  SHX/THX PUMP/1(FLOW FRACTION) -> [pthx_flow_frac]
  SHX SEC MIXING/1(Ts_shx_mix) -> [Ts_out_shx]
  SHX/THX PUMP/2(HEAT TRANSFER FRACTION) -> [pthx_hA_frac]
  SHX PRIM MIXING/1(Tp_shx_mix) -> [Tp_out_shx]
  [Ts_shx5_out] -> SHX SEC MIXING/1(Ts_shx5)
  [Tp_shx5_out] -> SHX PRIM MIXING/1(Tp_shx5)
  [pthx_flow_frac] -> SHX SEC MIXING/3(s_flow_frac)
  [Ts_shx6_out] -> SHX SEC MIXING/2(Ts_shx6)
  [Tp_shx6_out] -> SHX PRIM MIXING/2(Tp_shx6)
  THX2 HEAT TRANSFER/1(THX3 TEMPERATURES) -> THX3 MATERIAL TRANSPORT/1(THX3 TEMPERATURES), Tp_thx2_out/1, Ts_thx2_out/1
  [pshx_hA_frac] -> PHX5 HEAT TRANSFER/6(SECONDARY HEAT TRANSFER FRACTION)
  [Tp_out_shx_del] -> PHX5 HEAT TRANSFER/2(SECONDARY FLUID INLET TEMPERATURE)
  [pshx_flow_frac] -> PHX5 HEAT TRANSFER/5(SECONDARY FLOW FRACTION)
  [fuel_hA_frac] -> PHX5 HEAT TRANSFER/4(PRIMARY HEAT TRANSFER FRACTION)
  [Tf_in] -> PHX5 HEAT TRANSFER/1(PRIMARY FLUID INLET TEMPERATURE)
  [fuel_flow_frac] -> PHX5 HEAT TRANSFER/3(PRIMARY FLOW FRACTION)
  [pshx_flow_frac] -> PHX6 HEAT TRANSFER/5(SECONDARY FLOW FRACTION)
  [fuel_hA_frac] -> PHX6 HEAT TRANSFER/4(PRIMARY HEAT TRANSFER FRACTION)
  [pshx_hA_frac] -> PHX6 HEAT TRANSFER/6(SECONDARY HEAT TRANSFER FRACTION)
  [Tf_in] -> PHX6 HEAT TRANSFER/1(PRIMARY FLUID INLET TEMPERATURE)
  [fuel_flow_frac] -> PHX6 HEAT TRANSFER/3(PRIMARY FLOW FRACTION)
  [Tp_out_shx_del] -> PHX6 HEAT TRANSFER/2(SECONDARY FLUID INLET TEMPERATURE)
  [fuel_flow_frac] -> VAR DELAY FUNC/1
  [Tp_out_phx] -> HX TO CORE/1
  HX TO CORE/1 -> [Tp_out_phx_del]
  VAR DELAY FUNC/1 -> HX TO CORE/2
  PHX TO SHX DELAY/1 -> [Ts_out_phx_del]
  [pshx_flow_frac] -> VAR DELAY FUNC1/1
  VAR DELAY FUNC1/1 -> PHX TO SHX DELAY/2
  [Ts_out_phx] -> PHX TO SHX DELAY/1
  [pshx_flow_frac] -> SHX5 HEAT TRANSFER/3(PRIMARY FLOW FRACTION)
  [pshx_hA_frac] -> SHX5 HEAT TRANSFER/4(PRIMARY HEAT TRANSFER FRACTION)
  [pthx_hA_frac] -> SHX5 HEAT TRANSFER/6(SECONDARY HEAT TRANSFER FRACTION)
  [Ts_out_phx_del] -> SHX5 HEAT TRANSFER/1(PRIMARY FLUID INLET TEMPERATURE)
  [pthx_flow_frac] -> SHX5 HEAT TRANSFER/5(SECONDARY FLOW FRACTION)
  [pthx_hA_frac] -> SHX6 HEAT TRANSFER/6(SECONDARY HEAT TRANSFER FRACTION)
  [pshx_hA_frac] -> SHX6 HEAT TRANSFER/4(PRIMARY HEAT TRANSFER FRACTION)
  [pshx_flow_frac] -> SHX6 HEAT TRANSFER/3(PRIMARY FLOW FRACTION)
  [pthx_flow_frac] -> SHX6 HEAT TRANSFER/5(SECONDARY FLOW FRACTION)
  [Ts_out_phx_del] -> SHX6 HEAT TRANSFER/1(PRIMARY FLUID INLET TEMPERATURE)
  VAR DELAY FUNC2/1 -> SHX TO PHX DELAY/2
  [Tp_out_shx] -> SHX TO PHX DELAY/1
  [pshx_flow_frac] -> VAR DELAY FUNC2/1
  SHX TO PHX DELAY/1 -> [Tp_out_shx_del]
  [Ts_out_shx] -> SHX TO PHX DELAY1/1
  SHX TO PHX DELAY1/1 -> [Ts_out_shx_del]
  [pthx_flow_frac] -> VAR DELAY FUNC3/1
  VAR DELAY FUNC3/1 -> SHX TO PHX DELAY1/2
  Constant1/1 -> THX2 HEAT TRANSFER/5(SECONDARY FLOW FRACTION)
  Constant2/1 -> THX2 HEAT TRANSFER/6(SECONDARY HEAT TRANSFER FRACTION)
  From45/1 -> THX2 HEAT TRANSFER/1(PRIMARY FLUID INLET TEMPERATURE)
  From28/1 -> THX2 HEAT TRANSFER/3(PRIMARY FLOW FRACTION)
  From30/1 -> THX2 HEAT TRANSFER/4(PRIMARY HEAT TRANSFER FRACTION)
  BOILER & REHEATER/1(Coolant Exit Temp) -> Goto23/1
  From15/1 -> BOILER & REHEATER/1(Coolant Inlet Temp)
  Fractional Power Demand (fractional)/1(Power Demand(frac)) -> To Workspace/1, BOILER & REHEATER/2(Power Demand (Frac))
  [T3_in] -> SHX5 HEAT TRANSFER/2(SECONDARY FLUID INLET TEMPERATURE)
  [T3_in] -> SHX6 HEAT TRANSFER/2(SECONDARY FLUID INLET TEMPERATURE)
  HX3 HITEC INLET/1 -> [T3_in]
  [Ts_out_shx_del] -> HX3 HITEC OUTLET/1
  [pthx_flow_frac] -> HX3 HITEC FLOW/1
  [pthx_hA_frac] -> HX3 HITEC HEAT TRANSFER/1
  [pshx_flow_frac] -> SHX PRIM MIXING/3(p_flow_frac)

== system MSDR_v1.1/HEAT EXCHANGERS/PRE BoP MIXING ==
  Tshx1 : Inport
  delay1 : Inport  Port=2
  Tshx2 : Inport  Port=3
  delay2 : Inport  Port=4
  Tshx3 : Inport  Port=5
  delay3 : Inport  Port=6
  Fcn : Fcn  Expr=u[2]*W_31/m_3m*(u[1] - u[7]) + u[4]*W_32/m_3m*(u[3] - u[7]) + u[6]*W_33/m_3m*(u[5] - u[7])
  Integrator : Integrator  InitialCondition=T3_out
  Mux : Mux  Inputs=7
  T3_out : Outport
  wires:
  Tshx1/1 -> Mux/1
  delay1/1 -> Mux/2
  Tshx2/1 -> Mux/3
  delay2/1 -> Mux/4
  Tshx3/1 -> Mux/5
  delay3/1 -> Mux/6
  Mux/1 -> Fcn/1
  Fcn/1 -> Integrator/1
  Integrator/1 -> T3_out/1, Mux/7

== system MSDR_v1.1/HEAT EXCHANGERS/PRE CORE MIXING ==
  Tphx1 : Inport
  delay1 : Inport  Port=2
  Tphx2 : Inport  Port=3
  delay2 : Inport  Port=4
  Tphx3 : Inport  Port=5
  delay3 : Inport  Port=6
  Fcn : Fcn  Expr=u[2]*W_f1/m_fm*(u[1] - u[7]) + u[4]*W_f2/m_fm*(u[3] - u[7]) + u[6]*W_f3/m_fm*(u[5] - u[7])
  Integrator : Integrator  InitialCondition=Tf_in
  Mux : Mux  Inputs=7
  Tf_out : Outport
  wires:
  Tphx1/1 -> Mux/1
  delay1/1 -> Mux/2
  Tphx2/1 -> Mux/3
  delay2/1 -> Mux/4
  Tphx3/1 -> Mux/5
  delay3/1 -> Mux/6
  Mux/1 -> Fcn/1
  Fcn/1 -> Integrator/1
  Integrator/1 -> Tf_out/1, Mux/7

== system MSDR_v1.1/BALANCE OF PLANT/POWER/FEEDWATER HEATER 1 - LOW-PRESSURE ==
  note: Enthalpy of feedwater heater 1
  note: Heat transfer rate in the feedwater heater 1
  STEAM FLOW RATE - LP TURBINE : Inport
  STEAM BLEED FLOW - LP TURBINE : Inport  Port=2
  FLOW from FWH2 : Inport  Port=3
  ENTHALPY - CONDENSER : Inport  Port=4
  H'_fwh : Integrator  InitialCondition=H_fwh1
  Mux : Mux  Inputs=7
      settings: DisplayOption=signals
  Q_fwh1 : Fcn  Expr=h_fwh1*(u[3] + u[2])
  To Workspace : ToWorkspace  VariableName=FWH1_mux  SampleTime=0.1
      settings: Save2DSignal=2-D array (concatenate along first dimension)
  Unit Delay1 : UnitDelay  InitialCondition=W_fw  SampleTime=-1
  Unit Delay7 : UnitDelay  InitialCondition=96.368  SampleTime=-1
  W_fw : Fcn  Expr=u[1] + u[2] + u[3]
  d(H'_fwh)/dt : Fcn  Expr=u[6]/(tau_fwh1*u[7]) + (u[4] - u[5])/tau_fwh1
  ENTHALPY - FWH1 : Outport
  FEEDWATER FLOW RATE : Outport  Port=2
  wires:
  STEAM FLOW RATE - LP TURBINE/1 -> Mux/1
  STEAM BLEED FLOW - LP TURBINE/1 -> Mux/2
  FLOW from FWH2/1 -> Mux/3
  Mux/1 -> To Workspace/1, W_fw/1, Q_fwh1/1, d(H'_fwh)/dt/1
  ENTHALPY - CONDENSER/1 -> Mux/4
  d(H'_fwh)/dt/1 -> H'_fwh/1
  H'_fwh/1 -> Mux/5, ENTHALPY - FWH1/1
  Q_fwh1/1 -> Unit Delay7/1
  Unit Delay7/1 -> Mux/6
  W_fw/1 -> Unit Delay1/1
  Unit Delay1/1 -> FEEDWATER FLOW RATE/1, Mux/7

== system MSDR_v1.1/BALANCE OF PLANT/POWER/FEEDWATER HEATER 2 - HIGH-PRESSURE ==
  note: Enthalpy of feedwater heater 2
  note: Heat transfer rate in the feedwater heater 2
  note: Flow to FWH1
  note: Temperature of feedwater after heating
  STEAM BLEED FLOW - HP TURBINE : Inport
  FLOW from MOISTURE SEPARATOR : Inport  Port=2
  FLOW from REHEATER : Inport  Port=3
  FLOW from MS to RH : Inport  Port=4
  FLOW from FWH1 : Inport  Port=5
  ENTHALPY - FWH1 : Inport  Port=6
  STEAM FLOW RATE - NOZZLE CHEST : Inport  Port=7
  H_fwh : Integrator  InitialCondition=H_fwh2
  Mux : Mux  Inputs=11
      settings: DisplayOption=signals
  Q_fwh2 : Fcn  Expr=h_fwh2*(u[1] + u[2] + u[3])
  T_fw : Integrator  InitialCondition=205.58
  To Workspace : ToWorkspace  VariableName=FWH2_mux  SampleTime=0.1
      settings: Save2DSignal=2-D array (concatenate along first dimension)
  Unit Delay7 : UnitDelay  InitialCondition=70.197  SampleTime=-1
  d(H_fwh)/dt : Fcn  Expr=u[9]/(tau_fwh2*u[5]) + (u[6] - u[8])/tau_fwh2
  d(T_fw)/dt : Fcn  Expr=(u[9]/(tau_fwh2*u[5]) + (u[6] - Cp_fw*u[11])/tau_fwh2) / Cp_fw
  d(w'_fwh)/dt : Fcn  Expr=(u[7] - u[4])/tau_rh2 + (u[3] - u[10])/tau_rh2
  w'_fwh : Integrator  InitialCondition=118.44
  ENTHALPY - FWH2 : Outport
  FLOW to FWH1 : Outport  Port=2
  FEEDWATER FLOW RATE : Outport  Port=3
  TEMPERATURE - FEEDWATER : Outport  Port=4
  wires:
  STEAM BLEED FLOW - HP TURBINE/1 -> Mux/1
  FLOW from MOISTURE SEPARATOR/1 -> Mux/2
  FLOW from REHEATER/1 -> Mux/3
  FLOW from MS to RH/1 -> Mux/4
  d(H_fwh)/dt/1 -> H_fwh/1
  H_fwh/1 -> Mux/8, ENTHALPY - FWH2/1
  Q_fwh2/1 -> Unit Delay7/1
  Unit Delay7/1 -> Mux/9
  FLOW from FWH1/1 -> FEEDWATER FLOW RATE/1, Mux/5
  ENTHALPY - FWH1/1 -> Mux/6
  STEAM FLOW RATE - NOZZLE CHEST/1 -> Mux/7
  d(w'_fwh)/dt/1 -> w'_fwh/1
  w'_fwh/1 -> Mux/10, FLOW to FWH1/1
  d(T_fw)/dt/1 -> T_fw/1
  T_fw/1 -> Mux/11, TEMPERATURE - FEEDWATER/1
  Mux/1 -> To Workspace/1, d(T_fw)/dt/1, d(w'_fwh)/dt/1, Q_fwh2/1, d(H_fwh)/dt/1

== system MSDR_v1.1/BALANCE OF PLANT/POWER/HIGH PRESSURE TURBINE ==
  note: Steam flow from HP turbine to moisture separator
  note: HP turbine bleed flow rate to feed water heater 2
  note: Enthalpy of steam at moisture separator
  note: Enthalpy of steam at isentropic endpoints from pressure P_nc
  STEAM FLOW RATE - NOZZLE CHEST : Inport
  STEAM ENTHALPY - NOZZLE CHEST : Inport  Port=2
  STEAM PRESSURE - NOZZLE CHEST : Inport  Port=3
  STEAM PRESSURE - REHEATER : Inport  Port=4
  H_hp : Fcn  Expr=(u[8] - u[2])*eta_hp_isen + u[2]
  H_hp_isen : Fcn  Expr=term1 + ce1*(u[4] - p1) - ce2*(u[4] - p1)^2 - ce3*(u[1] - p2)
  Mux : Mux  Inputs=8
      settings: DisplayOption=signals
  To Workspace : ToWorkspace  VariableName=HPT_mux  SampleTime=0.1
      settings: Save2DSignal=2-D array (concatenate along first dimension)
  Unit Delay1 : UnitDelay  InitialCondition=2.6201  SampleTime=-1
  Unit Delay2 : UnitDelay  InitialCondition=2.5111  SampleTime=-1
  Unit Delay3 : UnitDelay  InitialCondition=44.134  SampleTime=-1
  d(w''_2)/dt : Fcn  Expr=((u[1] - u[6]) - u[5])/tau_hp
  w''_2 : Integrator  InitialCondition=w_hp_out
  w_b_hp : Fcn  Expr=K_b_hp*u[1]
  STEAM FLOW RATE - HP TURBINE : Outport
  STEAM BLEED FLOW - HP TURBINE : Outport  Port=2
  STEAM ENTHALPY - HP TURBINE : Outport  Port=3
  wires:
  STEAM FLOW RATE - NOZZLE CHEST/1 -> Mux/1
  STEAM ENTHALPY - NOZZLE CHEST/1 -> Mux/2
  STEAM PRESSURE - NOZZLE CHEST/1 -> Mux/3
  STEAM PRESSURE - REHEATER/1 -> Mux/4
  d(w''_2)/dt/1 -> w''_2/1
  w_b_hp/1 -> Unit Delay3/1
  H_hp/1 -> Unit Delay1/1
  H_hp_isen/1 -> Unit Delay2/1
  w''_2/1 -> STEAM FLOW RATE - HP TURBINE/1, Mux/5
  Mux/1 -> To Workspace/1, H_hp_isen/1, H_hp/1, w_b_hp/1, d(w''_2)/dt/1
  Unit Delay3/1 -> STEAM BLEED FLOW - HP TURBINE/1, Mux/6
  Unit Delay1/1 -> STEAM ENTHALPY - HP TURBINE/1, Mux/7
  Unit Delay2/1 -> Mux/8

== system MSDR_v1.1/BALANCE OF PLANT/POWER/LOW PRESSURE TURBINE ==
  note: Steam flow from HP turbine to moisture separator
  FLOW from REHEATER : Inport
  STEAM ENTHALPY - REHEATER : Inport  Port=2
  H_lp : Fcn  Expr=u[2] - eta_lp_isen*(u[2] - H_lp_isen)
  Mux : Mux  Inputs=5
      settings: DisplayOption=signals
  To Workspace : ToWorkspace  VariableName=LPT_mux  SampleTime=0.1
      settings: Save2DSignal=2-D array (concatenate along first dimension)
  Unit Delay1 : UnitDelay  InitialCondition=2.3089  SampleTime=-1
  Unit Delay3 : UnitDelay  InitialCondition=44.156  SampleTime=-1
  d(w'_3)/dt : Fcn  Expr=((u[1] - u[4]) - u[3])/tau_lp
  w'_3 : Integrator  InitialCondition=w_lp_out
  w_b_lp : Fcn  Expr=K_b_lp*u[1]
  STEAM FLOW RATE - LP TURBINE : Outport
  STEAM BLEED FLOW - LP TURBINE : Outport  Port=2
  STEAM ENTHALPY - LP TURBINE : Outport  Port=3
  wires:
  FLOW from REHEATER/1 -> Mux/1
  STEAM ENTHALPY - REHEATER/1 -> Mux/2
  w'_3/1 -> STEAM FLOW RATE - LP TURBINE/1, Mux/3
  d(w'_3)/dt/1 -> w'_3/1
  w_b_lp/1 -> Unit Delay3/1
  Mux/1 -> To Workspace/1, H_lp/1, w_b_lp/1, d(w'_3)/dt/1
  Unit Delay3/1 -> STEAM BLEED FLOW - LP TURBINE/1, Mux/4
  Unit Delay1/1 -> Mux/5, STEAM ENTHALPY - LP TURBINE/1
  H_lp/1 -> Unit Delay1/1

== system MSDR_v1.1/BALANCE OF PLANT/POWER/MOISTURE SEPARATOR ==
  note: Steam flow from moisture separator to reheater
  note: Steam flow from moisture separator to feedwater heater2
  ENTHALPY OF VAPORIZATION : Inport
  ENTHALPY OF REHEATER FEEDWATER : Inport  Port=2
  STEAM FLOW RATE - NOZZLE CHEST : Inport  Port=3
  STEAM FLOW RATE - HP TURBINE : Inport  Port=4
  STEAM BLEED FLOW - HP TURBINE : Inport  Port=5
  STEAM ENTHALPY - HP TURBINE : Inport  Port=6
  Mux : Mux  Inputs=8
      settings: DisplayOption=signals
  To Workspace : ToWorkspace  VariableName=MS_mux  SampleTime=0.1
      settings: Save2DSignal=2-D array (concatenate along first dimension)
  w'_2 : Fcn  Expr=(u[6] - u[2])/u[1] * u[4]
  w_ms : Fcn  Expr=(u[3] - u[5]) - u[8]
  FLOW to HEATER2 : Outport
  FLOW to REHEATER : Outport  Port=2
  wires:
  ENTHALPY OF VAPORIZATION/1 -> Mux/1
  ENTHALPY OF REHEATER FEEDWATER/1 -> Mux/2
  STEAM FLOW RATE - NOZZLE CHEST/1 -> Mux/3
  STEAM FLOW RATE - HP TURBINE/1 -> Mux/4
  STEAM BLEED FLOW - HP TURBINE/1 -> Mux/5
  STEAM ENTHALPY - HP TURBINE/1 -> Mux/6
  Mux/1 -> w'_2/1, w_ms/1, To Workspace/1
  w_ms/1 -> FLOW to HEATER2/1, Mux/7
  w'_2/1 -> FLOW to REHEATER/1, Mux/8

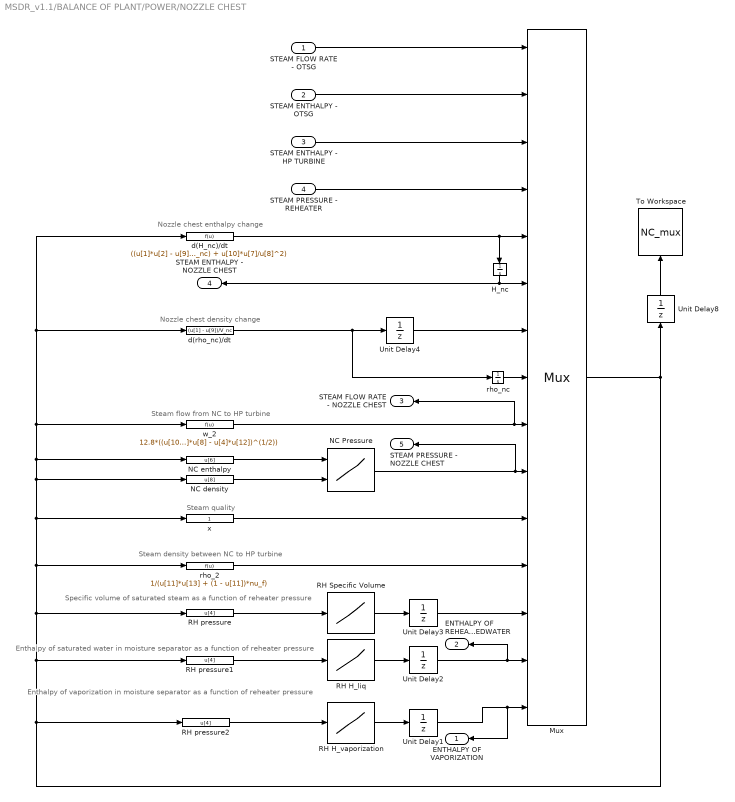
== system MSDR_v1.1/BALANCE OF PLANT/POWER/NOZZLE CHEST ==
  note: Nozzle chest density change
  note: Nozzle chest enthalpy change
  note: Steam flow from NC to HP turbine
  note: Steam quality
  note: Steam density between NC to HP turbine
  note: Specific volume of saturated steam as a function of reheater pressure
  note: Enthalpy of saturated water in moisture separator as a function of reheater pressure
  note: Enthalpy of vaporization in moisture separator as a function of reheater pressure
  STEAM FLOW RATE - OTSG : Inport
  STEAM ENTHALPY - OTSG : Inport  Port=2
  STEAM ENTHALPY - HP TURBINE : Inport  Port=3
  STEAM PRESSURE - REHEATER : Inport  Port=4
  H_nc : Integrator  InitialCondition=H_nc
  Mux : Mux  Inputs=15
      settings: DisplayOption=signals
  NC Pressure : Lookup_n-D  BreakpointsForDimension1=H_table  BreakpointsForDimension2=rho_table  Table=P_nc_table  InternalRulePriority=Speed  RndMeth=Simplest  InputSameDT=on
  NC density : Fcn  Expr=u[8]
  NC enthalpy : Fcn  Expr=u[6]
  RH H_liq : Lookup_n-D  NumberOfTableDimensions=1  BreakpointsForDimension1=P_rh_table1  Table=H_rh_table  InternalRulePriority=Speed  RndMeth=Simplest  InputSameDT=on
  RH H_vaporization : Lookup_n-D  NumberOfTableDimensions=1  BreakpointsForDimension1=P_rh_table1  Table=H_rhvap_table  InternalRulePriority=Speed  RndMeth=Simplest  InputSameDT=on
  RH Specific Volume : Lookup_n-D  NumberOfTableDimensions=1  BreakpointsForDimension1=P_rh_table1  Table=SV_nc_table  InternalRulePriority=Speed  RndMeth=Simplest  InputSameDT=on
  RH pressure : Fcn  Expr=u[4]
  RH pressure1 : Fcn  Expr=u[4]
  RH pressure2 : Fcn  Expr=u[4]
  To Workspace : ToWorkspace  VariableName=NC_mux  SampleTime=-1
      settings: Save2DSignal=2-D array (concatenate along first dimension)
  Unit Delay1 : UnitDelay  InitialCondition=1.8077  SampleTime=-1
  Unit Delay2 : UnitDelay  InitialCondition=.99522  SampleTime=-1
  Unit Delay3 : UnitDelay  InitialCondition=0.070431  SampleTime=-1
  Unit Delay4 : UnitDelay  SampleTime=-1
  Unit Delay8 : UnitDelay  InitialCondition=266.6348  SampleTime=-1
  d(H_nc)/dt : Fcn  Expr=((u[1]*u[2] - u[9]*u[6])/(u[8]*V_nc) + u[10]*u[7]/u[8]^2)
  d(rho_nc)/dt : Fcn  Expr=(u[1] - u[9])/V_nc
  rho_2 : Fcn  Expr=1/(u[11]*u[13] + (1 - u[11])*nu_f)
  rho_nc : Integrator  InitialCondition=74.07  UpperSaturationLimit=rho_nc
  w_2 : Fcn  Expr=12.8*((u[10]*u[8] - u[4]*u[12])^(1/2))
  x : Fcn  Expr=1
  ENTHALPY OF VAPORIZATION : Outport
  ENTHALPY OF REHEATER FEEDWATER : Outport  Port=2
  STEAM FLOW RATE - NOZZLE CHEST : Outport  Port=3
  STEAM ENTHALPY - NOZZLE CHEST : Outport  Port=4
  STEAM PRESSURE - NOZZLE CHEST : Outport  Port=5
  wires:
  STEAM FLOW RATE - OTSG/1 -> Mux/1
  STEAM ENTHALPY - OTSG/1 -> Mux/2
  STEAM ENTHALPY - HP TURBINE/1 -> Mux/3
  STEAM PRESSURE - REHEATER/1 -> Mux/4
  H_nc/1 -> Mux/6, STEAM ENTHALPY - NOZZLE CHEST/1
  NC density/1 -> NC Pressure/2
  NC enthalpy/1 -> NC Pressure/1
  x/1 -> Mux/11
  Mux/1 -> RH pressure2/1, RH pressure1/1, RH pressure/1, rho_2/1, x/1, NC density/1, NC enthalpy/1, w_2/1, d(rho_nc)/dt/1, d(H_nc)/dt/1, Unit Delay8/1
  d(H_nc)/dt/1 -> Mux/5, H_nc/1
  w_2/1 -> STEAM FLOW RATE - NOZZLE CHEST/1, Mux/9
  NC Pressure/1 -> STEAM PRESSURE - NOZZLE CHEST/1, Mux/10
  Unit Delay8/1 -> To Workspace/1
  RH pressure2/1 -> RH H_vaporization/1
  RH pressure1/1 -> RH H_liq/1
  RH Specific Volume/1 -> Unit Delay3/1
  RH pressure/1 -> RH Specific Volume/1
  RH H_liq/1 -> Unit Delay2/1
  RH H_vaporization/1 -> Unit Delay1/1
  Unit Delay1/1 -> ENTHALPY OF VAPORIZATION/1, Mux/15
  rho_nc/1 -> Mux/8
  Unit Delay2/1 -> ENTHALPY OF REHEATER FEEDWATER/1, Mux/14
  Unit Delay3/1 -> Mux/13
  rho_2/1 -> Mux/12
  d(rho_nc)/dt/1 -> Unit Delay4/1, rho_nc/1
  Unit Delay4/1 -> Mux/7
